simulink model "test_mdl_NI"  (R2018a)
settings: Solver=VariableStepAuto  StartTime=0.0  StopTime=10.0  RelTol=1e-3
(part 21 of 24)

== system test_mdl_NI/To_NI_HIL/SRR_L/RL_SOD/SRR_RL_001 ==
  in : Inport
  SRR_RL_CAN_DET_AMPLITUDE_01 : Subsystem
  SRR_RL_CAN_DET_AZIMUTH_01 : Subsystem
  SRR_RL_CAN_DET_ELEVATION_01 : Subsystem
  SRR_RL_CAN_DET_RANGE_01 : Subsystem
  SRR_RL_CAN_DET_RANGE_RATE_01 : Subsystem
  SRR_RL_CAN_DET_SUPER_RES_TARGET_01 : Subsystem
  SRR_RL_CAN_DET_VALID_LEVEL_01 : Subsystem
  bus_creator : BusCreator  Inputs=7
  bus_selector : BusSelector  OutputSignals=SRR_RL_CAN_DET_RANGE_01,SRR_RL_CAN_DET_RANGE_RATE_01,SRR_RL_CAN_DET_AZIMUTH_01,SRR_RL_CAN_DET_ELEVATION_01,SRR_RL_CAN_DET_SUPER_RES_TARGET_01,SRR_RL_CAN_DET_AMPLITUDE_01,SRR_RL_CAN_DET_VALID_LEVEL_01
  out_port : Outport
  wires:
  bus_creator/1 -> out_port/1  "SRR_RL_001"
  SRR_RL_CAN_DET_RANGE_01/1(out) -> bus_creator/1  "SRR_RL_CAN_DET_RANGE_01"
  SRR_RL_CAN_DET_RANGE_RATE_01/1(out) -> bus_creator/2  "SRR_RL_CAN_DET_RANGE_RATE_01"
  SRR_RL_CAN_DET_AZIMUTH_01/1(out) -> bus_creator/3  "SRR_RL_CAN_DET_AZIMUTH_01"
  SRR_RL_CAN_DET_ELEVATION_01/1(out) -> bus_creator/4  "SRR_RL_CAN_DET_ELEVATION_01"
  SRR_RL_CAN_DET_SUPER_RES_TARGET_01/1(out) -> bus_creator/5  "SRR_RL_CAN_DET_SUPER_RES_TARGET_01"
  SRR_RL_CAN_DET_AMPLITUDE_01/1(out) -> bus_creator/6  "SRR_RL_CAN_DET_AMPLITUDE_01"
  SRR_RL_CAN_DET_VALID_LEVEL_01/1(out) -> bus_creator/7  "SRR_RL_CAN_DET_VALID_LEVEL_01"
  bus_selector/1 -> SRR_RL_CAN_DET_RANGE_01/1(in)  "<SRR_RL_CAN_DET_RANGE_01>"
  bus_selector/2 -> SRR_RL_CAN_DET_RANGE_RATE_01/1(in)  "<SRR_RL_CAN_DET_RANGE_RATE_01>"
  bus_selector/3 -> SRR_RL_CAN_DET_AZIMUTH_01/1(in)  "<SRR_RL_CAN_DET_AZIMUTH_01>"
  bus_selector/4 -> SRR_RL_CAN_DET_ELEVATION_01/1(in)  "<SRR_RL_CAN_DET_ELEVATION_01>"
  bus_selector/5 -> SRR_RL_CAN_DET_SUPER_RES_TARGET_01/1(in)  "<SRR_RL_CAN_DET_SUPER_RES_TARGET_01>"
  bus_selector/6 -> SRR_RL_CAN_DET_AMPLITUDE_01/1(in)  "<SRR_RL_CAN_DET_AMPLITUDE_01>"
  bus_selector/7 -> SRR_RL_CAN_DET_VALID_LEVEL_01/1(in)  "<SRR_RL_CAN_DET_VALID_LEVEL_01>"
  in/1 -> bus_selector/1

== system test_mdl_NI/To_NI_HIL/SRR_L/RL_SOD/SRR_RL_002 ==
  in : Inport
  SRR_RL_CAN_DET_AMPLITUDE_02 : Subsystem
  SRR_RL_CAN_DET_AZIMUTH_02 : Subsystem
  SRR_RL_CAN_DET_ELEVATION_02 : Subsystem
  SRR_RL_CAN_DET_RANGE_02 : Subsystem
  SRR_RL_CAN_DET_RANGE_RATE_02 : Subsystem
  SRR_RL_CAN_DET_SUPER_RES_TARGET_02 : Subsystem
  SRR_RL_CAN_DET_VALID_LEVEL_02 : Subsystem
  bus_creator : BusCreator  Inputs=7
  bus_selector : BusSelector  OutputSignals=SRR_RL_CAN_DET_RANGE_02,SRR_RL_CAN_DET_RANGE_RATE_02,SRR_RL_CAN_DET_AZIMUTH_02,SRR_RL_CAN_DET_ELEVATION_02,SRR_RL_CAN_DET_SUPER_RES_TARGET_02,SRR_RL_CAN_DET_AMPLITUDE_02,SRR_RL_CAN_DET_VALID_LEVEL_02
  out_port : Outport
  wires:
  bus_creator/1 -> out_port/1  "SRR_RL_002"
  SRR_RL_CAN_DET_RANGE_02/1(out) -> bus_creator/1  "SRR_RL_CAN_DET_RANGE_02"
  SRR_RL_CAN_DET_RANGE_RATE_02/1(out) -> bus_creator/2  "SRR_RL_CAN_DET_RANGE_RATE_02"
  SRR_RL_CAN_DET_AZIMUTH_02/1(out) -> bus_creator/3  "SRR_RL_CAN_DET_AZIMUTH_02"
  SRR_RL_CAN_DET_ELEVATION_02/1(out) -> bus_creator/4  "SRR_RL_CAN_DET_ELEVATION_02"
  SRR_RL_CAN_DET_SUPER_RES_TARGET_02/1(out) -> bus_creator/5  "SRR_RL_CAN_DET_SUPER_RES_TARGET_02"
  SRR_RL_CAN_DET_AMPLITUDE_02/1(out) -> bus_creator/6  "SRR_RL_CAN_DET_AMPLITUDE_02"
  SRR_RL_CAN_DET_VALID_LEVEL_02/1(out) -> bus_creator/7  "SRR_RL_CAN_DET_VALID_LEVEL_02"
  bus_selector/1 -> SRR_RL_CAN_DET_RANGE_02/1(in)  "<SRR_RL_CAN_DET_RANGE_02>"
  bus_selector/2 -> SRR_RL_CAN_DET_RANGE_RATE_02/1(in)  "<SRR_RL_CAN_DET_RANGE_RATE_02>"
  bus_selector/3 -> SRR_RL_CAN_DET_AZIMUTH_02/1(in)  "<SRR_RL_CAN_DET_AZIMUTH_02>"
  bus_selector/4 -> SRR_RL_CAN_DET_ELEVATION_02/1(in)  "<SRR_RL_CAN_DET_ELEVATION_02>"
  bus_selector/5 -> SRR_RL_CAN_DET_SUPER_RES_TARGET_02/1(in)  "<SRR_RL_CAN_DET_SUPER_RES_TARGET_02>"
  bus_selector/6 -> SRR_RL_CAN_DET_AMPLITUDE_02/1(in)  "<SRR_RL_CAN_DET_AMPLITUDE_02>"
  bus_selector/7 -> SRR_RL_CAN_DET_VALID_LEVEL_02/1(in)  "<SRR_RL_CAN_DET_VALID_LEVEL_02>"
  in/1 -> bus_selector/1

== system test_mdl_NI/To_NI_HIL/SRR_L/RL_SOD/SRR_RL_003 ==
  in : Inport
  SRR_RL_CAN_DET_AMPLITUDE_03 : Subsystem
  SRR_RL_CAN_DET_AZIMUTH_03 : Subsystem
  SRR_RL_CAN_DET_ELEVATION_03 : Subsystem
  SRR_RL_CAN_DET_RANGE_03 : Subsystem
  SRR_RL_CAN_DET_RANGE_RATE_03 : Subsystem
  SRR_RL_CAN_DET_SUPER_RES_TARGET_03 : Subsystem
  SRR_RL_CAN_DET_VALID_LEVEL_03 : Subsystem
  bus_creator : BusCreator  Inputs=7
  bus_selector : BusSelector  OutputSignals=SRR_RL_CAN_DET_RANGE_03,SRR_RL_CAN_DET_RANGE_RATE_03,SRR_RL_CAN_DET_AZIMUTH_03,SRR_RL_CAN_DET_ELEVATION_03,SRR_RL_CAN_DET_SUPER_RES_TARGET_03,SRR_RL_CAN_DET_AMPLITUDE_03,SRR_RL_CAN_DET_VALID_LEVEL_03
  out_port : Outport
  wires:
  bus_creator/1 -> out_port/1  "SRR_RL_003"
  SRR_RL_CAN_DET_RANGE_03/1(out) -> bus_creator/1  "SRR_RL_CAN_DET_RANGE_03"
  SRR_RL_CAN_DET_RANGE_RATE_03/1(out) -> bus_creator/2  "SRR_RL_CAN_DET_RANGE_RATE_03"
  SRR_RL_CAN_DET_AZIMUTH_03/1(out) -> bus_creator/3  "SRR_RL_CAN_DET_AZIMUTH_03"
  SRR_RL_CAN_DET_ELEVATION_03/1(out) -> bus_creator/4  "SRR_RL_CAN_DET_ELEVATION_03"
  SRR_RL_CAN_DET_SUPER_RES_TARGET_03/1(out) -> bus_creator/5  "SRR_RL_CAN_DET_SUPER_RES_TARGET_03"
  SRR_RL_CAN_DET_AMPLITUDE_03/1(out) -> bus_creator/6  "SRR_RL_CAN_DET_AMPLITUDE_03"
  SRR_RL_CAN_DET_VALID_LEVEL_03/1(out) -> bus_creator/7  "SRR_RL_CAN_DET_VALID_LEVEL_03"
  bus_selector/1 -> SRR_RL_CAN_DET_RANGE_03/1(in)  "<SRR_RL_CAN_DET_RANGE_03>"
  bus_selector/2 -> SRR_RL_CAN_DET_RANGE_RATE_03/1(in)  "<SRR_RL_CAN_DET_RANGE_RATE_03>"
  bus_selector/3 -> SRR_RL_CAN_DET_AZIMUTH_03/1(in)  "<SRR_RL_CAN_DET_AZIMUTH_03>"
  bus_selector/4 -> SRR_RL_CAN_DET_ELEVATION_03/1(in)  "<SRR_RL_CAN_DET_ELEVATION_03>"
  bus_selector/5 -> SRR_RL_CAN_DET_SUPER_RES_TARGET_03/1(in)  "<SRR_RL_CAN_DET_SUPER_RES_TARGET_03>"
  bus_selector/6 -> SRR_RL_CAN_DET_AMPLITUDE_03/1(in)  "<SRR_RL_CAN_DET_AMPLITUDE_03>"
  bus_selector/7 -> SRR_RL_CAN_DET_VALID_LEVEL_03/1(in)  "<SRR_RL_CAN_DET_VALID_LEVEL_03>"
  in/1 -> bus_selector/1

== system test_mdl_NI/To_NI_HIL/SRR_R/FR_SOD/SRR_FR_001 ==
  in : Inport
  SRR_FR_CAN_DET_AMPLITUDE_01 : Subsystem
  SRR_FR_CAN_DET_AZIMUTH_01 : Subsystem
  SRR_FR_CAN_DET_ELEVATION_01 : Subsystem
  SRR_FR_CAN_DET_RANGE_01 : Subsystem
  SRR_FR_CAN_DET_RANGE_RATE_01 : Subsystem
  SRR_FR_CAN_DET_SUPER_RES_TARGET_01 : Subsystem
  SRR_FR_CAN_DET_VALID_LEVEL_01 : Subsystem
  bus_creator : BusCreator  Inputs=7
  bus_selector : BusSelector  OutputSignals=SRR_FR_CAN_DET_RANGE_01,SRR_FR_CAN_DET_RANGE_RATE_01,SRR_FR_CAN_DET_AZIMUTH_01,SRR_FR_CAN_DET_ELEVATION_01,SRR_FR_CAN_DET_SUPER_RES_TARGET_01,SRR_FR_CAN_DET_AMPLITUDE_01,SRR_FR_CAN_DET_VALID_LEVEL_01
  out_port : Outport
  wires:
  bus_creator/1 -> out_port/1  "SRR_FR_001"
  SRR_FR_CAN_DET_RANGE_01/1(out) -> bus_creator/1  "SRR_FR_CAN_DET_RANGE_01"
  SRR_FR_CAN_DET_RANGE_RATE_01/1(out) -> bus_creator/2  "SRR_FR_CAN_DET_RANGE_RATE_01"
  SRR_FR_CAN_DET_AZIMUTH_01/1(out) -> bus_creator/3  "SRR_FR_CAN_DET_AZIMUTH_01"
  SRR_FR_CAN_DET_ELEVATION_01/1(out) -> bus_creator/4  "SRR_FR_CAN_DET_ELEVATION_01"
  SRR_FR_CAN_DET_SUPER_RES_TARGET_01/1(out) -> bus_creator/5  "SRR_FR_CAN_DET_SUPER_RES_TARGET_01"
  SRR_FR_CAN_DET_AMPLITUDE_01/1(out) -> bus_creator/6  "SRR_FR_CAN_DET_AMPLITUDE_01"
  SRR_FR_CAN_DET_VALID_LEVEL_01/1(out) -> bus_creator/7  "SRR_FR_CAN_DET_VALID_LEVEL_01"
  bus_selector/1 -> SRR_FR_CAN_DET_RANGE_01/1(in)  "<SRR_FR_CAN_DET_RANGE_01>"
  bus_selector/2 -> SRR_FR_CAN_DET_RANGE_RATE_01/1(in)  "<SRR_FR_CAN_DET_RANGE_RATE_01>"
  bus_selector/3 -> SRR_FR_CAN_DET_AZIMUTH_01/1(in)  "<SRR_FR_CAN_DET_AZIMUTH_01>"
  bus_selector/4 -> SRR_FR_CAN_DET_ELEVATION_01/1(in)  "<SRR_FR_CAN_DET_ELEVATION_01>"
  bus_selector/5 -> SRR_FR_CAN_DET_SUPER_RES_TARGET_01/1(in)  "<SRR_FR_CAN_DET_SUPER_RES_TARGET_01>"
  bus_selector/6 -> SRR_FR_CAN_DET_AMPLITUDE_01/1(in)  "<SRR_FR_CAN_DET_AMPLITUDE_01>"
  bus_selector/7 -> SRR_FR_CAN_DET_VALID_LEVEL_01/1(in)  "<SRR_FR_CAN_DET_VALID_LEVEL_01>"
  in/1 -> bus_selector/1

== system test_mdl_NI/To_NI_HIL/SRR_R/FR_SOD/SRR_FR_002 ==
  in : Inport
  SRR_FR_CAN_DET_AMPLITUDE_02 : Subsystem
  SRR_FR_CAN_DET_AZIMUTH_02 : Subsystem
  SRR_FR_CAN_DET_ELEVATION_02 : Subsystem
  SRR_FR_CAN_DET_RANGE_02 : Subsystem
  SRR_FR_CAN_DET_RANGE_RATE_02 : Subsystem
  SRR_FR_CAN_DET_SUPER_RES_TARGET_02 : Subsystem
  SRR_FR_CAN_DET_VALID_LEVEL_02 : Subsystem
  bus_creator : BusCreator  Inputs=7
  bus_selector : BusSelector  OutputSignals=SRR_FR_CAN_DET_RANGE_02,SRR_FR_CAN_DET_RANGE_RATE_02,SRR_FR_CAN_DET_AZIMUTH_02,SRR_FR_CAN_DET_ELEVATION_02,SRR_FR_CAN_DET_SUPER_RES_TARGET_02,SRR_FR_CAN_DET_AMPLITUDE_02,SRR_FR_CAN_DET_VALID_LEVEL_02
  out_port : Outport
  wires:
  bus_creator/1 -> out_port/1  "SRR_FR_002"
  SRR_FR_CAN_DET_RANGE_02/1(out) -> bus_creator/1  "SRR_FR_CAN_DET_RANGE_02"
  SRR_FR_CAN_DET_RANGE_RATE_02/1(out) -> bus_creator/2  "SRR_FR_CAN_DET_RANGE_RATE_02"
  SRR_FR_CAN_DET_AZIMUTH_02/1(out) -> bus_creator/3  "SRR_FR_CAN_DET_AZIMUTH_02"
  SRR_FR_CAN_DET_ELEVATION_02/1(out) -> bus_creator/4  "SRR_FR_CAN_DET_ELEVATION_02"
  SRR_FR_CAN_DET_SUPER_RES_TARGET_02/1(out) -> bus_creator/5  "SRR_FR_CAN_DET_SUPER_RES_TARGET_02"
  SRR_FR_CAN_DET_AMPLITUDE_02/1(out) -> bus_creator/6  "SRR_FR_CAN_DET_AMPLITUDE_02"
  SRR_FR_CAN_DET_VALID_LEVEL_02/1(out) -> bus_creator/7  "SRR_FR_CAN_DET_VALID_LEVEL_02"
  bus_selector/1 -> SRR_FR_CAN_DET_RANGE_02/1(in)  "<SRR_FR_CAN_DET_RANGE_02>"
  bus_selector/2 -> SRR_FR_CAN_DET_RANGE_RATE_02/1(in)  "<SRR_FR_CAN_DET_RANGE_RATE_02>"
  bus_selector/3 -> SRR_FR_CAN_DET_AZIMUTH_02/1(in)  "<SRR_FR_CAN_DET_AZIMUTH_02>"
  bus_selector/4 -> SRR_FR_CAN_DET_ELEVATION_02/1(in)  "<SRR_FR_CAN_DET_ELEVATION_02>"
  bus_selector/5 -> SRR_FR_CAN_DET_SUPER_RES_TARGET_02/1(in)  "<SRR_FR_CAN_DET_SUPER_RES_TARGET_02>"
  bus_selector/6 -> SRR_FR_CAN_DET_AMPLITUDE_02/1(in)  "<SRR_FR_CAN_DET_AMPLITUDE_02>"
  bus_selector/7 -> SRR_FR_CAN_DET_VALID_LEVEL_02/1(in)  "<SRR_FR_CAN_DET_VALID_LEVEL_02>"
  in/1 -> bus_selector/1

== system test_mdl_NI/To_NI_HIL/SRR_R/FR_SOD/SRR_FR_003 ==
  in : Inport
  SRR_FR_CAN_DET_AMPLITUDE_03 : Subsystem
  SRR_FR_CAN_DET_AZIMUTH_03 : Subsystem
  SRR_FR_CAN_DET_ELEVATION_03 : Subsystem
  SRR_FR_CAN_DET_RANGE_03 : Subsystem
  SRR_FR_CAN_DET_RANGE_RATE_03 : Subsystem
  SRR_FR_CAN_DET_SUPER_RES_TARGET_03 : Subsystem
  SRR_FR_CAN_DET_VALID_LEVEL_03 : Subsystem
  bus_creator : BusCreator  Inputs=7
  bus_selector : BusSelector  OutputSignals=SRR_FR_CAN_DET_RANGE_03,SRR_FR_CAN_DET_RANGE_RATE_03,SRR_FR_CAN_DET_AZIMUTH_03,SRR_FR_CAN_DET_ELEVATION_03,SRR_FR_CAN_DET_SUPER_RES_TARGET_03,SRR_FR_CAN_DET_AMPLITUDE_03,SRR_FR_CAN_DET_VALID_LEVEL_03
  out_port : Outport
  wires:
  bus_creator/1 -> out_port/1  "SRR_FR_003"
  SRR_FR_CAN_DET_RANGE_03/1(out) -> bus_creator/1  "SRR_FR_CAN_DET_RANGE_03"
  SRR_FR_CAN_DET_RANGE_RATE_03/1(out) -> bus_creator/2  "SRR_FR_CAN_DET_RANGE_RATE_03"
  SRR_FR_CAN_DET_AZIMUTH_03/1(out) -> bus_creator/3  "SRR_FR_CAN_DET_AZIMUTH_03"
  SRR_FR_CAN_DET_ELEVATION_03/1(out) -> bus_creator/4  "SRR_FR_CAN_DET_ELEVATION_03"
  SRR_FR_CAN_DET_SUPER_RES_TARGET_03/1(out) -> bus_creator/5  "SRR_FR_CAN_DET_SUPER_RES_TARGET_03"
  SRR_FR_CAN_DET_AMPLITUDE_03/1(out) -> bus_creator/6  "SRR_FR_CAN_DET_AMPLITUDE_03"
  SRR_FR_CAN_DET_VALID_LEVEL_03/1(out) -> bus_creator/7  "SRR_FR_CAN_DET_VALID_LEVEL_03"
  bus_selector/1 -> SRR_FR_CAN_DET_RANGE_03/1(in)  "<SRR_FR_CAN_DET_RANGE_03>"
  bus_selector/2 -> SRR_FR_CAN_DET_RANGE_RATE_03/1(in)  "<SRR_FR_CAN_DET_RANGE_RATE_03>"
  bus_selector/3 -> SRR_FR_CAN_DET_AZIMUTH_03/1(in)  "<SRR_FR_CAN_DET_AZIMUTH_03>"
  bus_selector/4 -> SRR_FR_CAN_DET_ELEVATION_03/1(in)  "<SRR_FR_CAN_DET_ELEVATION_03>"
  bus_selector/5 -> SRR_FR_CAN_DET_SUPER_RES_TARGET_03/1(in)  "<SRR_FR_CAN_DET_SUPER_RES_TARGET_03>"
  bus_selector/6 -> SRR_FR_CAN_DET_AMPLITUDE_03/1(in)  "<SRR_FR_CAN_DET_AMPLITUDE_03>"
  bus_selector/7 -> SRR_FR_CAN_DET_VALID_LEVEL_03/1(in)  "<SRR_FR_CAN_DET_VALID_LEVEL_03>"
  in/1 -> bus_selector/1

== system test_mdl_NI/To_NI_HIL/SRR_R/RR_SOD/SRR_RR_001 ==
  in : Inport
  SRR_RR_CAN_DET_AMPLITUDE_01 : Subsystem
  SRR_RR_CAN_DET_AZIMUTH_01 : Subsystem
  SRR_RR_CAN_DET_ELEVATION_01 : Subsystem
  SRR_RR_CAN_DET_RANGE_01 : Subsystem
  SRR_RR_CAN_DET_RANGE_RATE_01 : Subsystem
  SRR_RR_CAN_DET_SUPER_RES_TARGET_01 : Subsystem
  SRR_RR_CAN_DET_VALID_LEVEL_01 : Subsystem
  bus_creator : BusCreator  Inputs=7
  bus_selector : BusSelector  OutputSignals=SRR_RR_CAN_DET_RANGE_01,SRR_RR_CAN_DET_RANGE_RATE_01,SRR_RR_CAN_DET_AZIMUTH_01,SRR_RR_CAN_DET_ELEVATION_01,SRR_RR_CAN_DET_SUPER_RES_TARGET_01,SRR_RR_CAN_DET_AMPLITUDE_01,SRR_RR_CAN_DET_VALID_LEVEL_01
  out_port : Outport
  wires:
  bus_creator/1 -> out_port/1  "SRR_RR_001"
  SRR_RR_CAN_DET_RANGE_01/1(out) -> bus_creator/1  "SRR_RR_CAN_DET_RANGE_01"
  SRR_RR_CAN_DET_RANGE_RATE_01/1(out) -> bus_creator/2  "SRR_RR_CAN_DET_RANGE_RATE_01"
  SRR_RR_CAN_DET_AZIMUTH_01/1(out) -> bus_creator/3  "SRR_RR_CAN_DET_AZIMUTH_01"
  SRR_RR_CAN_DET_ELEVATION_01/1(out) -> bus_creator/4  "SRR_RR_CAN_DET_ELEVATION_01"
  SRR_RR_CAN_DET_SUPER_RES_TARGET_01/1(out) -> bus_creator/5  "SRR_RR_CAN_DET_SUPER_RES_TARGET_01"
  SRR_RR_CAN_DET_AMPLITUDE_01/1(out) -> bus_creator/6  "SRR_RR_CAN_DET_AMPLITUDE_01"
  SRR_RR_CAN_DET_VALID_LEVEL_01/1(out) -> bus_creator/7  "SRR_RR_CAN_DET_VALID_LEVEL_01"
  bus_selector/1 -> SRR_RR_CAN_DET_RANGE_01/1(in)  "<SRR_RR_CAN_DET_RANGE_01>"
  bus_selector/2 -> SRR_RR_CAN_DET_RANGE_RATE_01/1(in)  "<SRR_RR_CAN_DET_RANGE_RATE_01>"
  bus_selector/3 -> SRR_RR_CAN_DET_AZIMUTH_01/1(in)  "<SRR_RR_CAN_DET_AZIMUTH_01>"
  bus_selector/4 -> SRR_RR_CAN_DET_ELEVATION_01/1(in)  "<SRR_RR_CAN_DET_ELEVATION_01>"
  bus_selector/5 -> SRR_RR_CAN_DET_SUPER_RES_TARGET_01/1(in)  "<SRR_RR_CAN_DET_SUPER_RES_TARGET_01>"
  bus_selector/6 -> SRR_RR_CAN_DET_AMPLITUDE_01/1(in)  "<SRR_RR_CAN_DET_AMPLITUDE_01>"
  bus_selector/7 -> SRR_RR_CAN_DET_VALID_LEVEL_01/1(in)  "<SRR_RR_CAN_DET_VALID_LEVEL_01>"
  in/1 -> bus_selector/1

== system test_mdl_NI/To_NI_HIL/SRR_R/RR_SOD/SRR_RR_002 ==
  in : Inport
  SRR_RR_CAN_DET_AMPLITUDE_02 : Subsystem
  SRR_RR_CAN_DET_AZIMUTH_02 : Subsystem
  SRR_RR_CAN_DET_ELEVATION_02 : Subsystem
  SRR_RR_CAN_DET_RANGE_02 : Subsystem
  SRR_RR_CAN_DET_RANGE_RATE_02 : Subsystem
  SRR_RR_CAN_DET_SUPER_RES_TARGET_02 : Subsystem
  SRR_RR_CAN_DET_VALID_LEVEL_02 : Subsystem
  bus_creator : BusCreator  Inputs=7
  bus_selector : BusSelector  OutputSignals=SRR_RR_CAN_DET_RANGE_02,SRR_RR_CAN_DET_RANGE_RATE_02,SRR_RR_CAN_DET_AZIMUTH_02,SRR_RR_CAN_DET_ELEVATION_02,SRR_RR_CAN_DET_SUPER_RES_TARGET_02,SRR_RR_CAN_DET_AMPLITUDE_02,SRR_RR_CAN_DET_VALID_LEVEL_02
  out_port : Outport
  wires:
  bus_creator/1 -> out_port/1  "SRR_RR_002"
  SRR_RR_CAN_DET_RANGE_02/1(out) -> bus_creator/1  "SRR_RR_CAN_DET_RANGE_02"
  SRR_RR_CAN_DET_RANGE_RATE_02/1(out) -> bus_creator/2  "SRR_RR_CAN_DET_RANGE_RATE_02"
  SRR_RR_CAN_DET_AZIMUTH_02/1(out) -> bus_creator/3  "SRR_RR_CAN_DET_AZIMUTH_02"
  SRR_RR_CAN_DET_ELEVATION_02/1(out) -> bus_creator/4  "SRR_RR_CAN_DET_ELEVATION_02"
  SRR_RR_CAN_DET_SUPER_RES_TARGET_02/1(out) -> bus_creator/5  "SRR_RR_CAN_DET_SUPER_RES_TARGET_02"
  SRR_RR_CAN_DET_AMPLITUDE_02/1(out) -> bus_creator/6  "SRR_RR_CAN_DET_AMPLITUDE_02"
  SRR_RR_CAN_DET_VALID_LEVEL_02/1(out) -> bus_creator/7  "SRR_RR_CAN_DET_VALID_LEVEL_02"
  bus_selector/1 -> SRR_RR_CAN_DET_RANGE_02/1(in)  "<SRR_RR_CAN_DET_RANGE_02>"
  bus_selector/2 -> SRR_RR_CAN_DET_RANGE_RATE_02/1(in)  "<SRR_RR_CAN_DET_RANGE_RATE_02>"
  bus_selector/3 -> SRR_RR_CAN_DET_AZIMUTH_02/1(in)  "<SRR_RR_CAN_DET_AZIMUTH_02>"
  bus_selector/4 -> SRR_RR_CAN_DET_ELEVATION_02/1(in)  "<SRR_RR_CAN_DET_ELEVATION_02>"
  bus_selector/5 -> SRR_RR_CAN_DET_SUPER_RES_TARGET_02/1(in)  "<SRR_RR_CAN_DET_SUPER_RES_TARGET_02>"
  bus_selector/6 -> SRR_RR_CAN_DET_AMPLITUDE_02/1(in)  "<SRR_RR_CAN_DET_AMPLITUDE_02>"
  bus_selector/7 -> SRR_RR_CAN_DET_VALID_LEVEL_02/1(in)  "<SRR_RR_CAN_DET_VALID_LEVEL_02>"
  in/1 -> bus_selector/1

== system test_mdl_NI/To_NI_HIL/SRR_R/RR_SOD/SRR_RR_003 ==
  in : Inport
  SRR_RR_CAN_DET_AMPLITUDE_03 : Subsystem
  SRR_RR_CAN_DET_AZIMUTH_03 : Subsystem
  SRR_RR_CAN_DET_ELEVATION_03 : Subsystem
  SRR_RR_CAN_DET_RANGE_03 : Subsystem
  SRR_RR_CAN_DET_RANGE_RATE_03 : Subsystem
  SRR_RR_CAN_DET_SUPER_RES_TARGET_03 : Subsystem
  SRR_RR_CAN_DET_VALID_LEVEL_03 : Subsystem
  bus_creator : BusCreator  Inputs=7
  bus_selector : BusSelector  OutputSignals=SRR_RR_CAN_DET_RANGE_03,SRR_RR_CAN_DET_RANGE_RATE_03,SRR_RR_CAN_DET_AZIMUTH_03,SRR_RR_CAN_DET_ELEVATION_03,SRR_RR_CAN_DET_SUPER_RES_TARGET_03,SRR_RR_CAN_DET_AMPLITUDE_03,SRR_RR_CAN_DET_VALID_LEVEL_03
  out_port : Outport
  wires:
  bus_creator/1 -> out_port/1  "SRR_RR_003"
  SRR_RR_CAN_DET_RANGE_03/1(out) -> bus_creator/1  "SRR_RR_CAN_DET_RANGE_03"
  SRR_RR_CAN_DET_RANGE_RATE_03/1(out) -> bus_creator/2  "SRR_RR_CAN_DET_RANGE_RATE_03"
  SRR_RR_CAN_DET_AZIMUTH_03/1(out) -> bus_creator/3  "SRR_RR_CAN_DET_AZIMUTH_03"
  SRR_RR_CAN_DET_ELEVATION_03/1(out) -> bus_creator/4  "SRR_RR_CAN_DET_ELEVATION_03"
  SRR_RR_CAN_DET_SUPER_RES_TARGET_03/1(out) -> bus_creator/5  "SRR_RR_CAN_DET_SUPER_RES_TARGET_03"
  SRR_RR_CAN_DET_AMPLITUDE_03/1(out) -> bus_creator/6  "SRR_RR_CAN_DET_AMPLITUDE_03"
  SRR_RR_CAN_DET_VALID_LEVEL_03/1(out) -> bus_creator/7  "SRR_RR_CAN_DET_VALID_LEVEL_03"
  bus_selector/1 -> SRR_RR_CAN_DET_RANGE_03/1(in)  "<SRR_RR_CAN_DET_RANGE_03>"
  bus_selector/2 -> SRR_RR_CAN_DET_RANGE_RATE_03/1(in)  "<SRR_RR_CAN_DET_RANGE_RATE_03>"
  bus_selector/3 -> SRR_RR_CAN_DET_AZIMUTH_03/1(in)  "<SRR_RR_CAN_DET_AZIMUTH_03>"
  bus_selector/4 -> SRR_RR_CAN_DET_ELEVATION_03/1(in)  "<SRR_RR_CAN_DET_ELEVATION_03>"
  bus_selector/5 -> SRR_RR_CAN_DET_SUPER_RES_TARGET_03/1(in)  "<SRR_RR_CAN_DET_SUPER_RES_TARGET_03>"
  bus_selector/6 -> SRR_RR_CAN_DET_AMPLITUDE_03/1(in)  "<SRR_RR_CAN_DET_AMPLITUDE_03>"
  bus_selector/7 -> SRR_RR_CAN_DET_VALID_LEVEL_03/1(in)  "<SRR_RR_CAN_DET_VALID_LEVEL_03>"
  in/1 -> bus_selector/1

== system test_mdl_NI/To_NI_HIL/Soft_ABS/ABS_BrkBst_Data/BrkTotTqRqDrv_No_Cnt ==
  in : Inport
  out : Outport
  wires:
  in/1 -> out/1

== system test_mdl_NI/To_NI_HIL/Soft_ABS/ABS_BrkBst_Data/BrkTotTqRqDrv_No_Cs ==
  in : Inport
  out : Outport
  wires:
  in/1 -> out/1

== system test_mdl_NI/To_NI_HIL/Soft_ABS/ABS_BrkBst_Data/BrkTot_Tq_RqDrv ==
  in : Inport
  out : Outport
  wires:
  in/1 -> out/1

== system test_mdl_NI/To_NI_HIL/Soft_ABS/Accel_Data/VehLat2_A_Actl ==
  in : Inport
  out : Outport
  wires:
  in/1 -> out/1

== system test_mdl_NI/To_NI_HIL/Soft_ABS/Accel_Data/VehLong2_A_Actl ==
  in : Inport
  out : Outport
  wires:
  in/1 -> out/1

== system test_mdl_NI/To_NI_HIL/Soft_ABS/BrakeSnData_3/VehLatComp_A_Actl ==
  in : Inport
  out : Outport
  wires:
  in/1 -> out/1

== system test_mdl_NI/To_NI_HIL/Soft_ABS/BrakeSnData_3/VehLongComp_A_Actl ==
  in : Inport
  out : Outport
  wires:
  in/1 -> out/1

== system test_mdl_NI/To_NI_HIL/Soft_ABS/BrakeSnData_3/VehOverGnd_V_Est ==
  in : Inport
  out : Outport
  wires:
  in/1 -> out/1

== system test_mdl_NI/To_NI_HIL/Soft_ABS/BrakeSnData_3/VehYawComp_W_Actl ==
  in : Inport
  out : Outport
  wires:
  in/1 -> out/1

== system test_mdl_NI/To_NI_HIL/Soft_ABS/BrakeSnData_4/BrkTot_Tq_Actl ==
  in : Inport
  out : Outport
  wires:
  in/1 -> out/1

== system test_mdl_NI/To_NI_HIL/Soft_ABS/BrakeSnData_4/VehRolComp_W_Actl ==
  in : Inport
  out : Outport
  wires:
  in/1 -> out/1

== system test_mdl_NI/To_NI_HIL/Soft_ABS/BrakeSnData_4/VehVertComp_A_Actl ==
  in : Inport
  out : Outport
  wires:
  in/1 -> out/1

== system test_mdl_NI/To_NI_HIL/Soft_ABS/BrakeSnData_5/SteWhlComp_An_Est ==
  in : Inport
  out : Outport
  wires:
  in/1 -> out/1

== system test_mdl_NI/To_NI_HIL/Soft_ABS/BrakeSysFeatures/VehVActlBrk_No_Cnt ==
  in : Inport
  out : Outport
  wires:
  in/1 -> out/1

== system test_mdl_NI/To_NI_HIL/Soft_ABS/BrakeSysFeatures/VehVActlBrk_No_Cs ==
  in : Inport
  out : Outport
  wires:
  in/1 -> out/1

== system test_mdl_NI/To_NI_HIL/Soft_ABS/BrakeSysFeatures/Veh_V_ActlBrk ==
  in : Inport
  out : Outport
  wires:
  in/1 -> out/1

== system test_mdl_NI/To_NI_HIL/Soft_ABS/BrakeSysFeatures_2/BpedMove_D_Actl ==
  in : Inport
  out : Outport
  wires:
  in/1 -> out/1

== system test_mdl_NI/To_NI_HIL/Soft_ABS/BrakeSysFeatures_2/BpedMove_No_Cnt ==
  in : Inport
  out : Outport
  wires:
  in/1 -> out/1

== system test_mdl_NI/To_NI_HIL/Soft_ABS/BrakeSysFeatures_2/BpedMove_No_Cs ==
  in : Inport
  out : Outport
  wires:
  in/1 -> out/1

== system test_mdl_NI/To_NI_HIL/Soft_ABS/DesiredTorqBrk/AccBrkActv_B_Actl ==
  in : Inport
  out : Outport
  wires:
  in/1 -> out/1

== system test_mdl_NI/To_NI_HIL/Soft_ABS/DesiredTorqBrk/AccBrkPrchgActv_B_Actl ==
  in : Inport
  out : Outport
  wires:
  in/1 -> out/1

== system test_mdl_NI/To_NI_HIL/Soft_ABS/DesiredTorqBrk/AccBrkTotTqMn_B_Actl ==
  in : Inport
  out : Outport
  wires:
  in/1 -> out/1

== system test_mdl_NI/To_NI_HIL/Soft_ABS/DesiredTorqBrk/AccStopActv_B_ActlBrk ==
  in : Inport
  out : Outport
  wires:
  in/1 -> out/1

== system test_mdl_NI/To_NI_HIL/Soft_ABS/DesiredTorqBrk/CmbbBaSensInc_B_Actl ==
  in : Inport
  out : Outport
  wires:
  in/1 -> out/1

== system test_mdl_NI/To_NI_HIL/Soft_ABS/DesiredTorqBrk/CmbbBrkDecel_B_Actl ==
  in : Inport
  out : Outport
  wires:
  in/1 -> out/1

== system test_mdl_NI/To_NI_HIL/Soft_ABS/DesiredTorqBrk/CmbbBrkPrchg_B_Actl ==
  in : Inport
  out : Outport
  wires:
  in/1 -> out/1

== system test_mdl_NI/To_NI_HIL/Soft_ABS/DesiredTorqBrk/VehLongOvrGnd_A_Est ==
  in : Inport
  out : Outport
  wires:
  in/1 -> out/1

== system test_mdl_NI/To_NI_HIL/Soft_ABS/DesiredTorqBrk/VehStop_D_Stat ==
  in : Inport
  out : Outport
  wires:
  in/1 -> out/1

== system test_mdl_NI/To_NI_HIL/Soft_ABS/DesiredTorqBrk/VehicleStationary ==
  in : Inport
  out : Outport
  wires:
  in/1 -> out/1

== system test_mdl_NI/To_NI_HIL/Soft_ABS/ToCarSim/MCPressure ==
  in : Inport
  out : Outport
  wires:
  in/1 -> out/1

== system test_mdl_NI/To_NI_HIL/Soft_ABS/WheelData/WhlDirRl_D_Actl ==
  in : Inport
  out : Outport
  wires:
  in/1 -> out/1

== system test_mdl_NI/To_NI_HIL/Soft_ABS/WheelData/WhlDirRr_D_Actl ==
  in : Inport
  out : Outport
  wires:
  in/1 -> out/1

== system test_mdl_NI/To_NI_HIL/Soft_ABS/WheelSpeed/WhlFl_W_Meas ==
  in : Inport
  out : Outport
  wires:
  in/1 -> out/1

== system test_mdl_NI/To_NI_HIL/Soft_ABS/WheelSpeed/WhlFr_W_Meas ==
  in : Inport
  out : Outport
  wires:
  in/1 -> out/1

== system test_mdl_NI/To_NI_HIL/Soft_ABS/WheelSpeed/WhlRl_W_Meas ==
  in : Inport
  out : Outport
  wires:
  in/1 -> out/1

== system test_mdl_NI/To_NI_HIL/Soft_ABS/WheelSpeed/WhlRotatFl_No_Cnt ==
  in : Inport
  out : Outport
  wires:
  in/1 -> out/1

== system test_mdl_NI/To_NI_HIL/Soft_ABS/WheelSpeed/WhlRotatFr_No_Cnt ==
  in : Inport
  out : Outport
  wires:
  in/1 -> out/1

== system test_mdl_NI/To_NI_HIL/Soft_ABS/WheelSpeed/WhlRotatRl_No_Cnt ==
  in : Inport
  out : Outport
  wires:
  in/1 -> out/1

== system test_mdl_NI/To_NI_HIL/Soft_ABS/WheelSpeed/WhlRotatRr_No_Cnt ==
  in : Inport
  out : Outport
  wires:
  in/1 -> out/1

== system test_mdl_NI/To_NI_HIL/Soft_ABS/WheelSpeed/WhlRr_W_Meas ==
  in : Inport
  out : Outport
  wires:
  in/1 -> out/1

== system test_mdl_NI/To_NI_HIL/Soft_ABS/Yaw_Data/VehYaw_W_Actl ==
  in : Inport
  out : Outport
  wires:
  in/1 -> out/1

== system test_mdl_NI/To_NI_HIL/Soft_BCM/BodyInfo_3/Ignition_Status ==
  in : Inport
  out : Outport
  wires:
  in/1 -> out/1

== system test_mdl_NI/To_NI_HIL/Soft_BCM/Cluster_Info1/OdometerMasterValue ==
  in : Inport
  out : Outport
  wires:
  in/1 -> out/1

== system test_mdl_NI/To_NI_HIL/Soft_BCM/Cluster_Info1/OdometerMasterValue_UB ==
  in : Inport
  out : Outport
  wires:
  in/1 -> out/1

== system test_mdl_NI/To_NI_HIL/Soft_BCM/GGCC_Config_Mgmt_ID/Byte_0 ==
  in : Inport
  out : Outport
  wires:
  in/1 -> out/1

== system test_mdl_NI/To_NI_HIL/Soft_BCM/GGCC_Config_Mgmt_ID/Byte_1 ==
  in : Inport
  out : Outport
  wires:
  in/1 -> out/1

== system test_mdl_NI/To_NI_HIL/Soft_BCM/GGCC_Config_Mgmt_ID/Byte_2 ==
  in : Inport
  out : Outport
  wires:
  in/1 -> out/1

== system test_mdl_NI/To_NI_HIL/Soft_BCM/GGCC_Config_Mgmt_ID/Byte_3 ==
  in : Inport
  out : Outport
  wires:
  in/1 -> out/1

== system test_mdl_NI/To_NI_HIL/Soft_BCM/GGCC_Config_Mgmt_ID/Byte_4 ==
  in : Inport
  out : Outport
  wires:
  in/1 -> out/1

== system test_mdl_NI/To_NI_HIL/Soft_BCM/GGCC_Config_Mgmt_ID/Byte_5 ==
  in : Inport
  out : Outport
  wires:
  in/1 -> out/1

== system test_mdl_NI/To_NI_HIL/Soft_BCM/GGCC_Config_Mgmt_ID/Byte_6 ==
  in : Inport
  out : Outport
  wires:
  in/1 -> out/1

== system test_mdl_NI/To_NI_HIL/Soft_BCM/GGCC_Config_Mgmt_ID/Byte_7 ==
  in : Inport
  out : Outport
  wires:
  in/1 -> out/1

== system test_mdl_NI/To_NI_HIL/Soft_BCM/Personality_BCM2_Data/RecallEvent_No_Cnt ==
  in : Inport
  out : Outport
  wires:
  in/1 -> out/1

== system test_mdl_NI/To_NI_HIL/Soft_ECM/EngBrakeData/ACCStopMde_D_Rq ==
  in : Inport
  out : Outport
  wires:
  in/1 -> out/1

== system test_mdl_NI/To_NI_HIL/Soft_ECM/EngBrakeData/Cc_Stat_D_Actl ==
  in : Inport
  out : Outport
  wires:
  in/1 -> out/1

== system test_mdl_NI/To_NI_HIL/Soft_ECM/EngBrakeData/CmbbEngTqMn_B_Rq ==
  in : Inport
  out : Outport
  wires:
  in/1 -> out/1

== system test_mdl_NI/To_NI_HIL/Soft_ECM/EngBrakeData/PrplTqMnSat_B_Actl ==
  in : Inport
  out : Outport
  wires:
  in/1 -> out/1

== system test_mdl_NI/To_NI_HIL/Soft_ECM/EngVehicleSpThrottle/EngAout_N_Actl ==
  in : Inport
  out : Outport
  wires:
  in/1 -> out/1

== system test_mdl_NI/To_NI_HIL/Soft_ECM/EngVehicleSpThrottle2/Veh_V_ActlEng ==
  in : Inport
  out : Outport
  wires:
  in/1 -> out/1

== system test_mdl_NI/To_NI_HIL/Soft_MRR/MRR_Detection/MRR_Detection_001 ==
  in : Inport
  CAN_DET_AMPLITUDE_01 : Subsystem
  CAN_DET_AZIMUTH_01 : Subsystem
  CAN_DET_RANGE_01 : Subsystem
  CAN_DET_RANGE_RATE_01 : Subsystem
  CAN_DET_VALID_LEVEL_01 : Subsystem
  bus_creator : BusCreator  Inputs=5
  bus_selector : BusSelector  OutputSignals=CAN_DET_RANGE_01,CAN_DET_RANGE_RATE_01,CAN_DET_AZIMUTH_01,CAN_DET_VALID_LEVEL_01,CAN_DET_AMPLITUDE_01
  out_port : Outport
  wires:
  bus_creator/1 -> out_port/1  "MRR_Detection_001"
  CAN_DET_RANGE_01/1(out) -> bus_creator/1  "CAN_DET_RANGE_01"
  CAN_DET_RANGE_RATE_01/1(out) -> bus_creator/2  "CAN_DET_RANGE_RATE_01"
  CAN_DET_AZIMUTH_01/1(out) -> bus_creator/3  "CAN_DET_AZIMUTH_01"
  CAN_DET_VALID_LEVEL_01/1(out) -> bus_creator/4  "CAN_DET_VALID_LEVEL_01"
  CAN_DET_AMPLITUDE_01/1(out) -> bus_creator/5  "CAN_DET_AMPLITUDE_01"
  bus_selector/1 -> CAN_DET_RANGE_01/1(in)  "<CAN_DET_RANGE_01>"
  bus_selector/2 -> CAN_DET_RANGE_RATE_01/1(in)  "<CAN_DET_RANGE_RATE_01>"
  bus_selector/3 -> CAN_DET_AZIMUTH_01/1(in)  "<CAN_DET_AZIMUTH_01>"
  bus_selector/4 -> CAN_DET_VALID_LEVEL_01/1(in)  "<CAN_DET_VALID_LEVEL_01>"
  bus_selector/5 -> CAN_DET_AMPLITUDE_01/1(in)  "<CAN_DET_AMPLITUDE_01>"
  in/1 -> bus_selector/1

== system test_mdl_NI/To_NI_HIL/Soft_MRR/MRR_Detection/MRR_Detection_002 ==
  in : Inport
  CAN_DET_AMPLITUDE_02 : Subsystem
  CAN_DET_AZIMUTH_02 : Subsystem
  CAN_DET_RANGE_02 : Subsystem
  CAN_DET_RANGE_RATE_02 : Subsystem
  CAN_DET_VALID_LEVEL_02 : Subsystem
  bus_creator : BusCreator  Inputs=5
  bus_selector : BusSelector  OutputSignals=CAN_DET_RANGE_02,CAN_DET_RANGE_RATE_02,CAN_DET_AZIMUTH_02,CAN_DET_VALID_LEVEL_02,CAN_DET_AMPLITUDE_02
  out_port : Outport
  wires:
  bus_creator/1 -> out_port/1  "MRR_Detection_002"
  CAN_DET_RANGE_02/1(out) -> bus_creator/1  "CAN_DET_RANGE_02"
  CAN_DET_RANGE_RATE_02/1(out) -> bus_creator/2  "CAN_DET_RANGE_RATE_02"
  CAN_DET_AZIMUTH_02/1(out) -> bus_creator/3  "CAN_DET_AZIMUTH_02"
  CAN_DET_VALID_LEVEL_02/1(out) -> bus_creator/4  "CAN_DET_VALID_LEVEL_02"
  CAN_DET_AMPLITUDE_02/1(out) -> bus_creator/5  "CAN_DET_AMPLITUDE_02"
  bus_selector/1 -> CAN_DET_RANGE_02/1(in)  "<CAN_DET_RANGE_02>"
  bus_selector/2 -> CAN_DET_RANGE_RATE_02/1(in)  "<CAN_DET_RANGE_RATE_02>"
  bus_selector/3 -> CAN_DET_AZIMUTH_02/1(in)  "<CAN_DET_AZIMUTH_02>"
  bus_selector/4 -> CAN_DET_VALID_LEVEL_02/1(in)  "<CAN_DET_VALID_LEVEL_02>"
  bus_selector/5 -> CAN_DET_AMPLITUDE_02/1(in)  "<CAN_DET_AMPLITUDE_02>"
  in/1 -> bus_selector/1

== system test_mdl_NI/To_NI_HIL/Soft_MRR/MRR_Detection/MRR_Detection_003 ==
  in : Inport
  CAN_DET_AMPLITUDE_03 : Subsystem
  CAN_DET_AZIMUTH_03 : Subsystem
  CAN_DET_RANGE_03 : Subsystem
  CAN_DET_RANGE_RATE_03 : Subsystem
  CAN_DET_VALID_LEVEL_03 : Subsystem
  bus_creator : BusCreator  Inputs=5
  bus_selector : BusSelector  OutputSignals=CAN_DET_RANGE_03,CAN_DET_RANGE_RATE_03,CAN_DET_AZIMUTH_03,CAN_DET_VALID_LEVEL_03,CAN_DET_AMPLITUDE_03
  out_port : Outport
  wires:
  bus_creator/1 -> out_port/1  "MRR_Detection_003"
  CAN_DET_RANGE_03/1(out) -> bus_creator/1  "CAN_DET_RANGE_03"
  CAN_DET_RANGE_RATE_03/1(out) -> bus_creator/2  "CAN_DET_RANGE_RATE_03"
  CAN_DET_AZIMUTH_03/1(out) -> bus_creator/3  "CAN_DET_AZIMUTH_03"
  CAN_DET_VALID_LEVEL_03/1(out) -> bus_creator/4  "CAN_DET_VALID_LEVEL_03"
  CAN_DET_AMPLITUDE_03/1(out) -> bus_creator/5  "CAN_DET_AMPLITUDE_03"
  bus_selector/1 -> CAN_DET_RANGE_03/1(in)  "<CAN_DET_RANGE_03>"
  bus_selector/2 -> CAN_DET_RANGE_RATE_03/1(in)  "<CAN_DET_RANGE_RATE_03>"
  bus_selector/3 -> CAN_DET_AZIMUTH_03/1(in)  "<CAN_DET_AZIMUTH_03>"
  bus_selector/4 -> CAN_DET_VALID_LEVEL_03/1(in)  "<CAN_DET_VALID_LEVEL_03>"
  bus_selector/5 -> CAN_DET_AMPLITUDE_03/1(in)  "<CAN_DET_AMPLITUDE_03>"
  in/1 -> bus_selector/1

== system test_mdl_NI/To_NI_HIL/Soft_PCM/EngBrakeData/BpedDrvAppl_D_Actl ==
  in : Inport
  out : Outport
  wires:
  in/1 -> out/1

== system test_mdl_NI/To_NI_HIL/Soft_PCM/EngBrakeData/BrkOnOffSwtch_D_Actl ==
  in : Inport
  out : Outport
  wires:
  in/1 -> out/1

== system test_mdl_NI/To_NI_HIL/Soft_PCM/EngVehicleSpThottle2/GearRvrse_D_Actl ==
  in : Inport
  out : Outport
  wires:
  in/1 -> out/1

== system test_mdl_NI/To_NI_HIL/Soft_PCM/EngVehicleSpThottle2/Veh_V_ActlEng ==
  in : Inport
  out : Outport
  wires:
  in/1 -> out/1

== system test_mdl_NI/To_NI_HIL/Soft_PCM/EngVehicleSpThottle2/Veh_V_RqCcSet ==
  in : Inport
  out : Outport
  wires:
  in/1 -> out/1

== system test_mdl_NI/To_NI_HIL/Soft_PCM/EngVehicleSpThrottle/ApedPosPcActl_No_Cs ==
  in : Inport
  out : Outport
  wires:
  in/1 -> out/1

== system test_mdl_NI/To_NI_HIL/Soft_PCM/EngVehicleSpThrottle/ApedPos_PcRate_ActlArb ==
  in : Inport
  out : Outport
  wires:
  in/1 -> out/1

== system test_mdl_NI/To_NI_HIL/Soft_PCM/EngVehicleSpThrottle/ApedPos_Pc_ActlArb ==
  in : Inport
  out : Outport
  wires:
  in/1 -> out/1

== system test_mdl_NI/To_NI_HIL/Soft_PCM/EngVehicleSpThrottle/ApedPos_Pc_ActlArb_No_Cnt ==
  in : Inport
  out : Outport
  wires:
  in/1 -> out/1

== system test_mdl_NI/To_NI_HIL/Soft_PCM/EngVehicleSpThrottle/EngAout_N_Actl ==
  in : Inport
  out : Outport
  wires:
  in/1 -> out/1

== system test_mdl_NI/To_NI_HIL/Soft_PCM/EngineClimateData/AirAmb_Te_Actl ==
  in : Inport
  out : Outport
  wires:
  in/1 -> out/1

== system test_mdl_NI/To_NI_HIL/Soft_PCM/EngineClimateData/AirAmb_Te_ActlFilt ==
  in : Inport
  out : Outport
  wires:
  in/1 -> out/1

== system test_mdl_NI/To_NI_HIL/Soft_PCM/EngineClimateData/EngAout_Aa_Actl ==
  in : Inport
  out : Outport
  wires:
  in/1 -> out/1

== system test_mdl_NI/To_NI_HIL/Soft_PCM/EngineClutchData/CluPdlPosPcMeas_D_Qf ==
  in : Inport
  out : Outport
  wires:
  in/1 -> out/1

== system test_mdl_NI/To_NI_HIL/Soft_PCM/EngineClutchData/CluPdlPos_Pc_Meas ==
  in : Inport
  out : Outport
  wires:
  in/1 -> out/1

== system test_mdl_NI/To_NI_HIL/Soft_PCM/EngineClutchData/CluPdl_PcRate_Actl ==
  in : Inport
  out : Outport
  wires:
  in/1 -> out/1

== system test_mdl_NI/To_NI_HIL/Soft_PCM/EngineData_7/FuelFlw_Vl_Dsply ==
  in : Inport
  out : Outport
  wires:
  in/1 -> out/1

== system test_mdl_NI/To_NI_HIL/Soft_PCM/EngineData_7/OdoCount ==
  in : Inport
  out : Outport
  wires:
  in/1 -> out/1

== system test_mdl_NI/To_NI_HIL/Soft_PCM/PowertrainData_10/GearLvr_D_ActlDrv ==
  in : Inport
  out : Outport
  wires:
  in/1 -> out/1

== system test_mdl_NI/To_NI_HIL/Soft_PCM/PowertrainData_10/GearPos_No_Cnt ==
  in : Inport
  out : Outport
  wires:
  in/1 -> out/1

== system test_mdl_NI/To_NI_HIL/Soft_PCM/PowertrainData_10/GearPos_No_Cs ==
  in : Inport
  out : Outport
  wires:
  in/1 -> out/1

== system test_mdl_NI/To_NI_HIL/Soft_PCM/TorqueDataEngFlags/PrplWhlTotTqRq_No_Cs ==
  in : Inport
  out : Outport
  wires:
  in/1 -> out/1

== system test_mdl_NI/To_NI_HIL/Soft_PCM/TorqueDataEngFlags/PrplWhlTot_Tq_Rq ==
  in : Inport
  out : Outport
  wires:
  in/1 -> out/1

== system test_mdl_NI/To_NI_HIL/Soft_PCM/TorqueDataEngFlags/PrplWhlTot_Tq_Rq_No_Cnt ==
  in : Inport
  out : Outport
  wires:
  in/1 -> out/1

== system test_mdl_NI/To_NI_HIL/Soft_PCM/VehicleOperatingModes/ElPw_D_Stat ==
  in : Inport
  out : Outport
  wires:
  in/1 -> out/1

== system test_mdl_NI/To_NI_HIL/Soft_PCM/VehicleOperatingModes/ElPw_D_StatStrtStop ==
  in : Inport
  out : Outport
  wires:
  in/1 -> out/1

== system test_mdl_NI/To_NI_HIL/Soft_PCM/VehicleOperatingModes/Eng_D_Stat ==
  in : Inport
  out : Outport
  wires:
  in/1 -> out/1

== system test_mdl_NI/To_NI_HIL/Soft_PCM/VehicleOperatingModes/PrplWhlTot2_Tq_Rq ==
  in : Inport
  out : Outport
  wires:
  in/1 -> out/1

== system test_mdl_NI/To_NI_HIL/Soft_PCM/VehicleOperatingModes/PwPckTq_D_Stat ==
  in : Inport
  out : Outport
  wires:
  in/1 -> out/1

== system test_mdl_NI/To_NI_HIL/Soft_RCM/Accel_Data/VehLat2_A_Actl ==
  in : Inport
  out : Outport
  wires:
  in/1 -> out/1

== system test_mdl_NI/To_NI_HIL/Soft_RCM/Accel_Data/VehLatAActl_D_Qf ==
  in : Inport
  out : Outport
  wires:
  in/1 -> out/1

== system test_mdl_NI/To_NI_HIL/Soft_RCM/Accel_Data/VehLatLongVert_No_Cnt ==
  in : Inport
  out : Outport
  wires:
  in/1 -> out/1

== system test_mdl_NI/To_NI_HIL/Soft_RCM/Accel_Data/VehLatLongVert_No_Cs ==
  in : Inport
  out : Outport
  wires:
  in/1 -> out/1

== system test_mdl_NI/To_NI_HIL/Soft_RCM/Accel_Data/VehLong2_A_Actl ==
  in : Inport
  out : Outport
  wires:
  in/1 -> out/1

== system test_mdl_NI/To_NI_HIL/Soft_RCM/Accel_Data/VehLongAActl_D_Qf ==
  in : Inport
  out : Outport
  wires:
  in/1 -> out/1

== system test_mdl_NI/To_NI_HIL/Soft_RCM/Accel_Data/VehVert2_A_Actl ==
  in : Inport
  out : Outport
  wires:
  in/1 -> out/1

== system test_mdl_NI/To_NI_HIL/Soft_RCM/Accel_Data/VehVertAActl_D_Qf ==
  in : Inport
  out : Outport
  wires:
  in/1 -> out/1

== system test_mdl_NI/To_NI_HIL/Soft_RCM/RCMStatusMessage2/FirstRowBuckleDriver ==
  in : Inport
  out : Outport
  wires:
  in/1 -> out/1

== system test_mdl_NI/To_NI_HIL/Soft_RCM/RCMStatusMessage2/RstrnImpactEvntStatus ==
  in : Inport
  out : Outport
  wires:
  in/1 -> out/1

== system test_mdl_NI/To_NI_HIL/Soft_RCM/Yaw_Data/VehRolWActl_D_Qf ==
  in : Inport
  out : Outport
  wires:
  in/1 -> out/1

== system test_mdl_NI/To_NI_HIL/Soft_RCM/Yaw_Data/VehRol_W_Actl ==
  in : Inport
  out : Outport
  wires:
  in/1 -> out/1

== system test_mdl_NI/To_NI_HIL/Soft_RCM/Yaw_Data/VehRollYawW_No_Cs ==
  in : Inport
  out : Outport
  wires:
  in/1 -> out/1

== system test_mdl_NI/To_NI_HIL/Soft_RCM/Yaw_Data/VehRollYaw_No_Cnt ==
  in : Inport
  out : Outport
  wires:
  in/1 -> out/1

== system test_mdl_NI/To_NI_HIL/Soft_RCM/Yaw_Data/VehYawWActl_D_Qf ==
  in : Inport
  out : Outport
  wires:
  in/1 -> out/1

== system test_mdl_NI/To_NI_HIL/Soft_RCM/Yaw_Data/VehYaw_W_Actl ==
  in : Inport
  out : Outport
  wires:
  in/1 -> out/1

== system test_mdl_NI/To_NI_HIL/Soft_SCCM/Steering_Data/AccButtnGapDecPress ==
  in : Inport
  out : Outport
  wires:
  in/1 -> out/1

== system test_mdl_NI/To_NI_HIL/Soft_SCCM/Steering_Data/AccButtnGapIncPress ==
  in : Inport
  out : Outport
  wires:
  in/1 -> out/1

== system test_mdl_NI/To_NI_HIL/Soft_SCCM/Steering_Data/AhbStat_B_Dsply ==
  in : Inport
  out : Outport
  wires:
  in/1 -> out/1

== system test_mdl_NI/To_NI_HIL/Soft_SCCM/Steering_Data/AslButtnOnOffCnclPress ==
  in : Inport
  out : Outport
  wires:
  in/1 -> out/1

== system test_mdl_NI/To_NI_HIL/Soft_SCCM/Steering_Data/AslButtnOnOffPress ==
  in : Inport
  out : Outport
  wires:
  in/1 -> out/1

== system test_mdl_NI/To_NI_HIL/Soft_SCCM/Steering_Data/CcAslButtnCnclPress ==
  in : Inport
  out : Outport
  wires:
  in/1 -> out/1

== system test_mdl_NI/To_NI_HIL/Soft_SCCM/Steering_Data/CcAslButtnCnclResPress ==
  in : Inport
  out : Outport
  wires:
  in/1 -> out/1

== system test_mdl_NI/To_NI_HIL/Soft_SCCM/Steering_Data/CcAslButtnOnPress ==
  in : Inport
  out : Outport
  wires:
  in/1 -> out/1

== system test_mdl_NI/To_NI_HIL/Soft_SCCM/Steering_Data/CcAslButtnResDecPress ==
  in : Inport
  out : Outport
  wires:
  in/1 -> out/1

== system test_mdl_NI/To_NI_HIL/Soft_SCCM/Steering_Data/CcAslButtnResIncPress ==
  in : Inport
  out : Outport
  wires:
  in/1 -> out/1

== system test_mdl_NI/To_NI_HIL/Soft_SCCM/Steering_Data/CcAslButtnSetDecPress ==
  in : Inport
  out : Outport
  wires:
  in/1 -> out/1

== system test_mdl_NI/To_NI_HIL/Soft_SCCM/Steering_Data/CcAslButtnSetIncPress ==
  in : Inport
  out : Outport
  wires:
  in/1 -> out/1

== system test_mdl_NI/To_NI_HIL/Soft_SCCM/Steering_Data/CcAslButtnSetPress ==
  in : Inport
  out : Outport
  wires:
  in/1 -> out/1

== system test_mdl_NI/To_NI_HIL/Soft_SCCM/Steering_Data/CcAsllButtnResPress ==
  in : Inport
  out : Outport
  wires:
  in/1 -> out/1

== system test_mdl_NI/To_NI_HIL/Soft_SCCM/Steering_Data/CcButtnOffPress ==
  in : Inport
  out : Outport
  wires:
  in/1 -> out/1

== system test_mdl_NI/To_NI_HIL/Soft_SCCM/Steering_Data/CcButtnOnOffCnclPress ==
  in : Inport
  out : Outport
  wires:
  in/1 -> out/1

== system test_mdl_NI/To_NI_HIL/Soft_SCCM/Steering_Data/CcButtnOnOffPress ==
  in : Inport
  out : Outport
  wires:
  in/1 -> out/1

== system test_mdl_NI/To_NI_HIL/Soft_SCCM/Steering_Data/CcButtnOnPress ==
  in : Inport
  out : Outport
  wires:
  in/1 -> out/1

== system test_mdl_NI/To_NI_HIL/Soft_SCCM/Steering_Data/HeadLghtHiCtrl_D_RqAhb ==
  in : Inport
  out : Outport
  wires:
  in/1 -> out/1

== system test_mdl_NI/To_NI_HIL/Soft_SCCM/Steering_Data/HeadLghtHiOn_B_StatAhb ==
  in : Inport
  out : Outport
  wires:
  in/1 -> out/1

== system test_mdl_NI/To_NI_HIL/Soft_SCCM/Steering_Wheel_Data2/SteWhlSwtchBack_B_Stat ==
  in : Inport
  out : Outport
  wires:
  in/1 -> out/1

== system test_mdl_NI/To_NI_HIL/Soft_SCCM/Steering_Wheel_Data2/SteWhlSwtchDown_B_Stat ==
  in : Inport
  out : Outport
  wires:
  in/1 -> out/1

== system test_mdl_NI/To_NI_HIL/Soft_SCCM/Steering_Wheel_Data2/SteWhlSwtchLeft_B_Stat ==
  in : Inport
  out : Outport
  wires:
  in/1 -> out/1

== system test_mdl_NI/To_NI_HIL/Soft_SCCM/Steering_Wheel_Data2/SteWhlSwtchMenu_B_Stat ==
  in : Inport
  out : Outport
  wires:
  in/1 -> out/1

== system test_mdl_NI/To_NI_HIL/Soft_SCCM/Steering_Wheel_Data2/SteWhlSwtchOk_B_Stat ==
  in : Inport
  out : Outport
  wires:
  in/1 -> out/1

== system test_mdl_NI/To_NI_HIL/Soft_SCCM/Steering_Wheel_Data2/SteWhlSwtchRght_B_Stat ==
  in : Inport
  out : Outport
  wires:
  in/1 -> out/1

== system test_mdl_NI/To_NI_HIL/Soft_SCCM/Steering_Wheel_Data2/SteWhlSwtchUp_B_Stat ==
  in : Inport
  out : Outport
  wires:
  in/1 -> out/1

== system test_mdl_NI/To_NI_HIL/Soft_TCM/TransGearData/GearLvrPos_D_Actl ==
  in : Inport
  out : Outport
  wires:
  in/1 -> out/1

== system test_mdl_NI/CAN_Signal/GWM/GSM/Gear_Shift_by_Wire_2_FD1_168/GearButtnStuck_B_Actl ==
  in : Inport
  out : Outport
  wires:
  in/1 -> out/1

== system test_mdl_NI/CAN_Signal/GWM/GSM/Gear_Shift_by_Wire_2_FD1_168/GsmSrvcRqd_B_Rq ==
  in : Inport
  out : Outport
  wires:
  in/1 -> out/1

== system test_mdl_NI/CAN_Signal/GWM/GSM/Gear_Shift_by_Wire_2_FD1_168/TrnGearPwmFalt_B_Actl ==
  in : Inport
  out : Outport
  wires:
  in/1 -> out/1

== system test_mdl_NI/CAN_Signal/GWM/GSM/Gear_Shift_by_Wire_2_FD1_168/TrnTrcmPwmSig_D_Actl ==
  in : Inport
  out : Outport
  wires:
  in/1 -> out/1

== system test_mdl_NI/CAN_Signal/GWM/GSM/Gear_Shift_by_Wire_FD1_5A/BrkSwtchPos_B_ActlGsm ==
  in : Inport
  out : Outport
  wires:
  in/1 -> out/1

== system test_mdl_NI/CAN_Signal/GWM/GSM/Gear_Shift_by_Wire_FD1_5A/DrQltyDrv_D_StatGsm ==
  in : Inport
  out : Outport
  wires:
  in/1 -> out/1

== system test_mdl_NI/CAN_Signal/GWM/GSM/Gear_Shift_by_Wire_FD1_5A/GsmGearMsgTxt_D_Rq ==
  in : Inport
  out : Outport
  wires:
  in/1 -> out/1

== system test_mdl_NI/CAN_Signal/GWM/GSM/Gear_Shift_by_Wire_FD1_5A/PrkBrkActv_D_RqGsmGear ==
  in : Inport
  out : Outport
  wires:
  in/1 -> out/1

== system test_mdl_NI/CAN_Signal/GWM/GSM/Gear_Shift_by_Wire_FD1_5A/TrnBtsiOvrrd_B_Stat ==
  in : Inport
  out : Outport
  wires:
  in/1 -> out/1

== system test_mdl_NI/CAN_Signal/GWM/GSM/Gear_Shift_by_Wire_FD1_5A/TrnGearButtn_B_ActlD0 ==
  in : Inport
  out : Outport
  wires:
  in/1 -> out/1

== system test_mdl_NI/CAN_Signal/GWM/GSM/Gear_Shift_by_Wire_FD1_5A/TrnGearButtn_B_ActlD1 ==
  in : Inport
  out : Outport
  wires:
  in/1 -> out/1

== system test_mdl_NI/CAN_Signal/GWM/GSM/Gear_Shift_by_Wire_FD1_5A/TrnGearButtn_B_ActlD2 ==
  in : Inport
  out : Outport
  wires:
  in/1 -> out/1

== system test_mdl_NI/CAN_Signal/GWM/GSM/Gear_Shift_by_Wire_FD1_5A/TrnGearButtn_B_ActlM0 ==
  in : Inport
  out : Outport
  wires:
  in/1 -> out/1

== system test_mdl_NI/CAN_Signal/GWM/GSM/Gear_Shift_by_Wire_FD1_5A/TrnGearButtn_B_ActlM1 ==
  in : Inport
  out : Outport
  wires:
  in/1 -> out/1

== system test_mdl_NI/CAN_Signal/GWM/GSM/Gear_Shift_by_Wire_FD1_5A/TrnGearButtn_B_ActlM2 ==
  in : Inport
  out : Outport
  wires:
  in/1 -> out/1

== system test_mdl_NI/CAN_Signal/GWM/GSM/Gear_Shift_by_Wire_FD1_5A/TrnGearButtn_B_ActlN0 ==
  in : Inport
  out : Outport
  wires:
  in/1 -> out/1

== system test_mdl_NI/CAN_Signal/GWM/GSM/Gear_Shift_by_Wire_FD1_5A/TrnGearButtn_B_ActlN1 ==
  in : Inport
  out : Outport
  wires:
  in/1 -> out/1

== system test_mdl_NI/CAN_Signal/GWM/GSM/Gear_Shift_by_Wire_FD1_5A/TrnGearButtn_B_ActlN2 ==
  in : Inport
  out : Outport
  wires:
  in/1 -> out/1

== system test_mdl_NI/CAN_Signal/GWM/GSM/Gear_Shift_by_Wire_FD1_5A/TrnGearButtn_B_ActlP0 ==
  in : Inport
  out : Outport
  wires:
  in/1 -> out/1

== system test_mdl_NI/CAN_Signal/GWM/GSM/Gear_Shift_by_Wire_FD1_5A/TrnGearButtn_B_ActlP1 ==
  in : Inport
  out : Outport
  wires:
  in/1 -> out/1

== system test_mdl_NI/CAN_Signal/GWM/GSM/Gear_Shift_by_Wire_FD1_5A/TrnGearButtn_B_ActlP2 ==
  in : Inport
  out : Outport
  wires:
  in/1 -> out/1

== system test_mdl_NI/CAN_Signal/GWM/GSM/Gear_Shift_by_Wire_FD1_5A/TrnGearButtn_B_ActlR0 ==
  in : Inport
  out : Outport
  wires:
  in/1 -> out/1

== system test_mdl_NI/CAN_Signal/GWM/GSM/Gear_Shift_by_Wire_FD1_5A/TrnGearButtn_B_ActlR1 ==
  in : Inport
  out : Outport
  wires:
  in/1 -> out/1

== system test_mdl_NI/CAN_Signal/GWM/GSM/Gear_Shift_by_Wire_FD1_5A/TrnGearButtn_B_ActlR2 ==
  in : Inport
  out : Outport
  wires:
  in/1 -> out/1

== system test_mdl_NI/CAN_Signal/GWM/GSM/Gear_Shift_by_Wire_FD1_5A/TrnGearButtn_U_Actl ==
  in : Inport
  out : Outport
  wires:
  in/1 -> out/1

== system test_mdl_NI/CAN_Signal/GWM/GSM/Gear_Shift_by_Wire_FD1_5A/TrnGearRqCnt_B_Actl ==
  in : Inport
  out : Outport
  wires:
  in/1 -> out/1

== system test_mdl_NI/CAN_Signal/GWM/GSM/Gear_Shift_by_Wire_FD1_5A/TrnGear_D_RqDrv ==
  in : Inport
  out : Outport
  wires:
  in/1 -> out/1

== system test_mdl_NI/CAN_Signal/GWM/GSM/Gear_Shift_by_Wire_FD1_5A/TrnGear_No_Cnt ==
  in : Inport
  out : Outport
  wires:
  in/1 -> out/1

== system test_mdl_NI/CAN_Signal/GWM/GSM/Gear_Shift_by_Wire_FD1_5A/TrnGear_No_Cs ==
  in : Inport
  out : Outport
  wires:
  in/1 -> out/1

== system test_mdl_NI/CAN_Signal/GWM/GSM/Gear_Shift_by_Wire_FD1_5A/TrnGsmNtmState_D_Actl ==
  in : Inport
  out : Outport
  wires:
  in/1 -> out/1

== system test_mdl_NI/CAN_Signal/GWM/GSM/Gear_Shift_by_Wire_FD1_5A/TrnRng_D_RqGsm ==
  in : Inport
  out : Outport
  wires:
  in/1 -> out/1

== system test_mdl_NI/CAN_Signal/GWM/GSM/Gear_Shift_by_Wire_FD1_5A/TrnValidGearRq_D_Stat ==
  in : Inport
  out : Outport
  wires:
  in/1 -> out/1

== system test_mdl_NI/CAN_Signal/GWM/Other_GWMTx/AC_Compressor_Data_FD1/ElCmprBattSysU_D_Falt ==
  in : Inport
  out : Outport
  wires:
  in/1 -> out/1

== system test_mdl_NI/CAN_Signal/GWM/Other_GWMTx/AC_Compressor_Data_FD1/ElCmprBattURng_D_Falt ==
  in : Inport
  out : Outport
  wires:
  in/1 -> out/1

== system test_mdl_NI/CAN_Signal/GWM/Other_GWMTx/AC_Compressor_Data_FD1/ElCmprInnrErr_D_Falt ==
  in : Inport
  out : Outport
  wires:
  in/1 -> out/1

== system test_mdl_NI/CAN_Signal/GWM/Other_GWMTx/AC_Compressor_Data_FD1/ElCmprLostComm_D_Falt ==
  in : Inport
  out : Outport
  wires:
  in/1 -> out/1

== system test_mdl_NI/CAN_Signal/GWM/Other_GWMTx/AC_Compressor_Data_FD1/ElCmprOverLoad_D_Falt ==
  in : Inport
  out : Outport
  wires:
  in/1 -> out/1

== system test_mdl_NI/CAN_Signal/GWM/Other_GWMTx/AC_Compressor_Data_FD1/ElCmprOverTe_D_Falt ==
  in : Inport
  out : Outport
  wires:
  in/1 -> out/1

== system test_mdl_NI/CAN_Signal/GWM/Other_GWMTx/AC_Compressor_Data_FD1/ElCmprOverTe_D_Stat ==
  in : Inport
  out : Outport
  wires:
  in/1 -> out/1

== system test_mdl_NI/CAN_Signal/GWM/Other_GWMTx/AC_Compressor_Data_FD1/ElCmprPerfErr_D_Falt ==
  in : Inport
  out : Outport
  wires:
  in/1 -> out/1

== system test_mdl_NI/CAN_Signal/GWM/Other_GWMTx/AC_Compressor_Data_FD1/ElCmprSysU_D_Falt ==
  in : Inport
  out : Outport
  wires:
  in/1 -> out/1

== system test_mdl_NI/CAN_Signal/GWM/Other_GWMTx/AC_Compressor_Data_FD1/ElCmprUHi_D_Stat ==
  in : Inport
  out : Outport
  wires:
  in/1 -> out/1

== system test_mdl_NI/CAN_Signal/GWM/Other_GWMTx/AC_Compressor_Data_FD1/ElCmprUHi_U_Actl ==
  in : Inport
  out : Outport
  wires:
  in/1 -> out/1

== system test_mdl_NI/CAN_Signal/GWM/Other_GWMTx/AC_Compressor_Data_FD1/ElCmpr_D_Stat ==
  in : Inport
  out : Outport
  wires:
  in/1 -> out/1

== system test_mdl_NI/CAN_Signal/GWM/Other_GWMTx/AC_Compressor_Data_FD1/ElCmpr_N_Actl ==
  in : Inport
  out : Outport
  wires:
  in/1 -> out/1

== system test_mdl_NI/CAN_Signal/GWM/Other_GWMTx/AC_Compressor_Data_FD1/ElCmpr_Pw_Actl ==
  in : Inport
  out : Outport
  wires:
  in/1 -> out/1

== system test_mdl_NI/CAN_Signal/GWM/Other_GWMTx/AC_Compressor_Req_FD1/ElCmprEnbl_B_Rq ==
  in : Inport
  out : Outport
  wires:
  in/1 -> out/1

== system test_mdl_NI/CAN_Signal/GWM/Other_GWMTx/AC_Compressor_Req_FD1/ElCmpr_N_Rq ==
  in : Inport
  out : Outport
  wires:
  in/1 -> out/1

== system test_mdl_NI/CAN_Signal/GWM/Other_GWMTx/APIMGPS_Data_Nav_1_FD1/GPS_Latitude_Degrees ==
  in : Inport
  out : Outport
  wires:
  in/1 -> out/1

== system test_mdl_NI/CAN_Signal/GWM/Other_GWMTx/APIMGPS_Data_Nav_1_FD1/GPS_Latitude_Min_dec ==
  in : Inport
  out : Outport
  wires:
  in/1 -> out/1

== system test_mdl_NI/CAN_Signal/GWM/Other_GWMTx/APIMGPS_Data_Nav_1_FD1/GPS_Latitude_Minutes ==
  in : Inport
  out : Outport
  wires:
  in/1 -> out/1

== system test_mdl_NI/CAN_Signal/GWM/Other_GWMTx/APIMGPS_Data_Nav_1_FD1/GPS_Longitude_Degrees ==
  in : Inport
  out : Outport
  wires:
  in/1 -> out/1

== system test_mdl_NI/CAN_Signal/GWM/Other_GWMTx/APIMGPS_Data_Nav_1_FD1/GPS_Longitude_Min_dec ==
  in : Inport
  out : Outport
  wires:
  in/1 -> out/1

== system test_mdl_NI/CAN_Signal/GWM/Other_GWMTx/APIMGPS_Data_Nav_1_FD1/GPS_Longitude_Minutes ==
  in : Inport
  out : Outport
  wires:
  in/1 -> out/1

== system test_mdl_NI/CAN_Signal/GWM/Other_GWMTx/APIMGPS_Data_Nav_1_FD1/GpsHsphLattSth_D_Actl ==
  in : Inport
  out : Outport
  wires:
  in/1 -> out/1

== system test_mdl_NI/CAN_Signal/GWM/Other_GWMTx/APIMGPS_Data_Nav_1_FD1/GpsHsphLongEast_D_Actl ==
  in : Inport
  out : Outport
  wires:
  in/1 -> out/1

== system test_mdl_NI/CAN_Signal/GWM/Other_GWMTx/APIMGPS_Data_Nav_2_FD1/GPS_Actual_vs_Infer_pos ==
  in : Inport
  out : Outport
  wires:
  in/1 -> out/1

== system test_mdl_NI/CAN_Signal/GWM/Other_GWMTx/APIMGPS_Data_Nav_2_FD1/GPS_Compass_direction ==
  in : Inport
  out : Outport
  wires:
  in/1 -> out/1

== system test_mdl_NI/CAN_Signal/GWM/Other_GWMTx/APIMGPS_Data_Nav_2_FD1/GPS_Pdop ==
  in : Inport
  out : Outport
  wires:
  in/1 -> out/1

== system test_mdl_NI/CAN_Signal/GWM/Other_GWMTx/APIMGPS_Data_Nav_2_FD1/GPS_UTC_hours ==
  in : Inport
  out : Outport
  wires:
  in/1 -> out/1

== system test_mdl_NI/CAN_Signal/GWM/Other_GWMTx/APIMGPS_Data_Nav_2_FD1/GPS_UTC_minutes ==
  in : Inport
  out : Outport
  wires:
  in/1 -> out/1

== system test_mdl_NI/CAN_Signal/GWM/Other_GWMTx/APIMGPS_Data_Nav_2_FD1/GPS_UTC_seconds ==
  in : Inport
  out : Outport
  wires:
  in/1 -> out/1

== system test_mdl_NI/CAN_Signal/GWM/Other_GWMTx/APIMGPS_Data_Nav_2_FD1/GpsUtcDay_No_Actl ==
  in : Inport
  out : Outport
  wires:
  in/1 -> out/1

== system test_mdl_NI/CAN_Signal/GWM/Other_GWMTx/APIMGPS_Data_Nav_2_FD1/GpsUtcMnth_No_Actl ==
  in : Inport
  out : Outport
  wires:
  in/1 -> out/1

== system test_mdl_NI/CAN_Signal/GWM/Other_GWMTx/APIMGPS_Data_Nav_2_FD1/GpsUtcYr_No_Actl ==
  in : Inport
  out : Outport
  wires:
  in/1 -> out/1

== system test_mdl_NI/CAN_Signal/GWM/Other_GWMTx/APIMGPS_Data_Nav_2_FD1/Gps_B_Falt ==
  in : Inport
  out : Outport
  wires:
  in/1 -> out/1

== system test_mdl_NI/CAN_Signal/GWM/Other_GWMTx/APIM_Request_Signals_1_FD1/ChrgOvrdExitScrn_D_Rq ==
  in : Inport
  out : Outport
  wires:
  in/1 -> out/1

== system test_mdl_NI/CAN_Signal/GWM/Other_GWMTx/APIM_Request_Signals_1_FD1/EmPrflButtnAssoc_D_Rq ==
  in : Inport
  out : Outport
  wires:
  in/1 -> out/1

== system test_mdl_NI/CAN_Signal/GWM/Other_GWMTx/APIM_Request_Signals_1_FD1/EmPrflKeyAssoc_D_Rq ==
  in : Inport
  out : Outport
  wires:
  in/1 -> out/1

== system test_mdl_NI/CAN_Signal/GWM/Other_GWMTx/APIM_Request_Signals_1_FD1/EmPrflNo_D_Rq ==
  in : Inport
  out : Outport
  wires:
  in/1 -> out/1

== system test_mdl_NI/CAN_Signal/GWM/Other_GWMTx/APIM_Request_Signals_1_FD1/Em_D_Stat ==
  in : Inport
  out : Outport
  wires:
  in/1 -> out/1

== system test_mdl_NI/CAN_Signal/GWM/Other_GWMTx/APIM_Request_Signals_1_FD1/Rba_D_Rq ==
  in : Inport
  out : Outport
  wires:
  in/1 -> out/1
